simulink model "SineWaveAdd_Project1"  (R2016b)
settings: Solver=VariableStepAuto  StartTime=0.0  StopTime=10.0  MaxStep=0.01  RelTol=1e-3
settings Model: Creator=1026691  LastModifiedBy=1026691

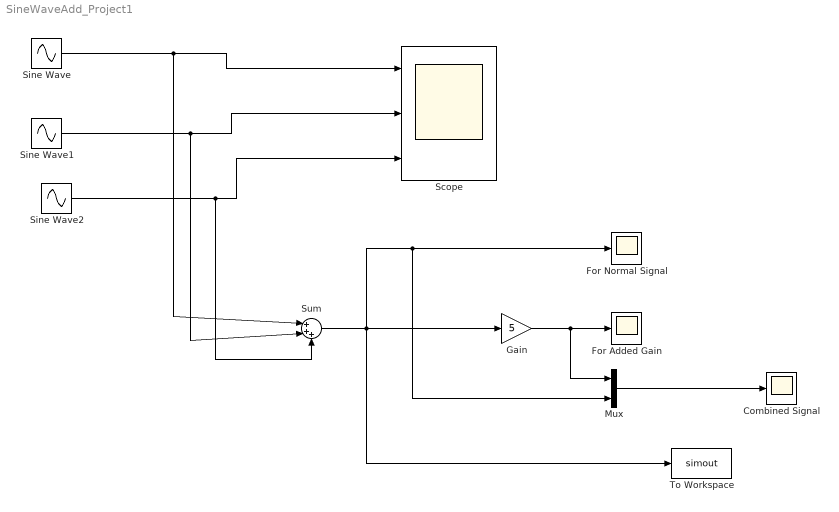
== system SineWaveAdd_Project1 ==
  "Combined Signal " : Scope
  For Added Gain : Scope
  For Normal Signal : Scope
  Gain : Gain  Gain=5
  Mux : Mux  Inputs=2
  Scope : Scope  NumInputPorts=3
  Sine Wave : Sin  Amplitude=3  SampleTime=0
  Sine Wave1 : Sin  Amplitude=5  Frequency=5  SampleTime=0
  Sine Wave2 : Sin  Amplitude=10  Frequency=10  SampleTime=0
  Sum : Sum  Inputs=|+++
  To Workspace : ToWorkspace  VariableName=simout  SaveFormat=Timeseries  SampleTime=-1
  wires:
  Sine Wave/1 -> Sum/1, Scope/1
  Sine Wave1/1 -> Sum/2, Scope/2
  Sine Wave2/1 -> Sum/3, Scope/3
  Sum/1 -> Gain/1, To Workspace/1, Mux/2, For Normal Signal/1
  Gain/1 -> Mux/1, For Added Gain/1
  Mux/1 -> "Combined Signal "/1
